simulink model "tr_frame_aided_correlator"  (Simulink 7.9)
settings: Solver=FixedStepDiscrete  SolverMode=SingleTasking  StartTime=0.0  StopTime=120  RelTol=1e-3
undefined symbols (not defined in the file): addr
libraries: shlslibv1 x27
settings Model: synDspstartup=OK  Creator=sszilvasi  LastModifiedBy=sszilvasi
settings DataIOCC: SaveOutput=off  SignalLogging=off  SaveTime=off
settings OptimizationCC: InlineParams=on
settings DebuggingCC: AlgebraicLoopMsg=error  InheritedTsInSrcMsg=none

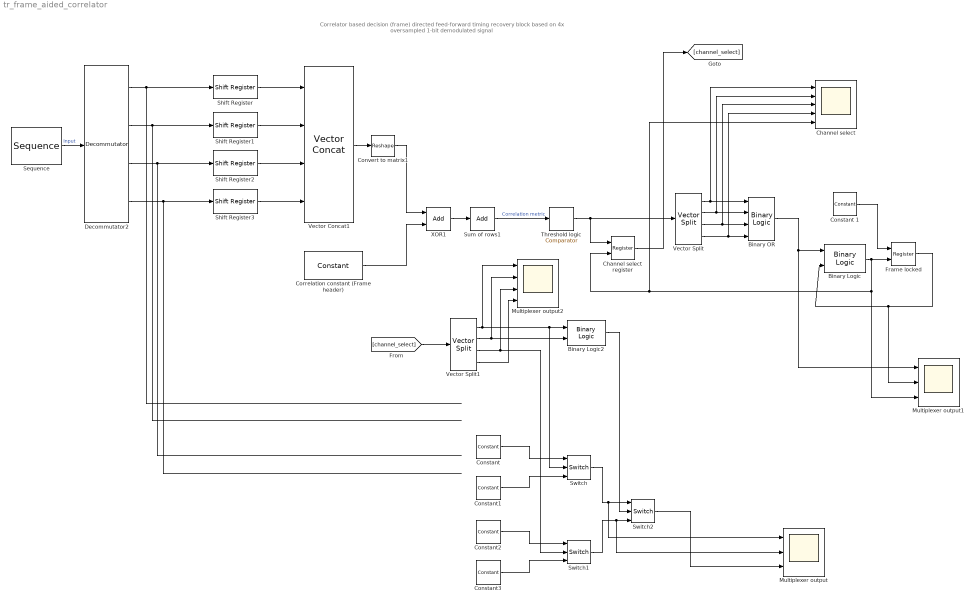
== system tr_frame_aided_correlator ==
  note: Correlator based decision (frame) directed feed-forward timing recovery block
      | based on 4x oversampled 1-bit demodulated signal
  Binary Logic : shlslibv1/Math Functions/Binary Logic  syn_binlog_exp=a&~b  synBlockType=primitive  synLatency=0  synBlockId=13
  Binary Logic2 : shlslibv1/Math Functions/Binary Logic  syn_binlog_exp=a|b  synBlockType=primitive  synLatency=0  synBlockId=13
  Binary OR : shlslibv1/Math Functions/Binary Logic  syn_binlog_exp=a|b|c|d  synBlockType=primitive  synLatency=0  synBlockId=13
  Channel select : Scope  NumInputPorts=5
      settings: YMin=-5~-5~-5~-5~-5  YMax=5~5~5~5~5
  Channel select register : shlslibv1/Memories/Register  syn_delay_val=1  syn_rst_port=off  syn_en_port=on  synBlockType=custom  synLatency=1
  Constant : shlslibv1/Sources/Constant  syn_cst_val=0  syn_cst_fl=0  syn_cst_dt=unsigned  syn_cst_rnd=on  syn_cst_st=-1  synBlockType=primitive  synLatency=0  synBlockId=15
  Constant 1 : shlslibv1/Sources/Constant  syn_cst_val=1  syn_cst_fl=0  syn_cst_dt=unsigned  syn_cst_rnd=on  syn_cst_st=-1  synBlockType=primitive  synLatency=0  synBlockId=15
  Constant1 : shlslibv1/Sources/Constant  syn_cst_val=1  syn_cst_fl=0  syn_cst_dt=unsigned  syn_cst_rnd=on  syn_cst_st=-1  synBlockType=primitive  synLatency=0  synBlockId=15
  Constant2 : shlslibv1/Sources/Constant  syn_cst_val=2  syn_cst_fl=0  syn_cst_dt=unsigned  syn_cst_rnd=on  syn_cst_st=-1  synBlockType=primitive  synLatency=0  synBlockId=15
  Constant3 : shlslibv1/Sources/Constant  syn_cst_val=3  syn_cst_fl=0  syn_cst_dt=unsigned  syn_cst_rnd=on  syn_cst_st=-1  synBlockType=primitive  synLatency=0  synBlockId=15
  Convert to matrix1 : shlslibv1/Signal Operations/Reshape  syn_op_dim_type=Specify  syn_op_dim=[4 4]  syn_ip_order=Column First  syn_op_order=Column First  syn_inh_port=off  synBlockType=primitive  synLatency=0  synBlockId=158
  Correlation constant (Frame header) : shlslibv1/Sources/Constant  syn_cst_val=[1 1 0 0]'*ones(1,4)  syn_cst_fl=0  syn_cst_dt=unsigned  syn_cst_rnd=on  syn_cst_st=-1  synBlockType=primitive  synLatency=0  synBlockId=15
  Decommutator2 : shlslibv1/Signal Operations/Decommutator  syn_outport_nb=4  syn_outport_vec=off  synBlockType=custom  synLatency=1
  Frame locked : shlslibv1/Memories/Register  syn_delay_val=1  syn_rst_port=off  syn_en_port=on  synBlockType=custom  synLatency=1
  Multiplexer output : Scope  NumInputPorts=3
      settings: YMin=-5~-5~-5  YMax=5~5~5
  Multiplexer output1 : Scope  NumInputPorts=3
      settings: YMin=-5~-5~-5  YMax=5~5~5  SaveName=ScopeData2
  Multiplexer output2 : Scope  NumInputPorts=4
      settings: YMin=-5~-5~-5~-5  YMax=5~5~5~5  SaveName=ScopeData3
  Sequence : shlslibv1/Sources/Sequence  syn_seq_vec=[zeros(1,8) 0 0 0 1 1 0 1 0 1]  syn_seq_wl=1  syn_seq_fl=0  syn_seq_dt=unsigned  syn_rst_port=off  syn_en_port=off  syn_seq_st=1  synBlockType=custom  synLatency=1
  Shift Register{,1..3} (4 alike) : shlslibv1/Memories/Shift Register  syn_shift_dynamic=off  syn_shift_vec=[0:3]  syn_shift_val=16  syn_vect_out=Merge to vector  syn_rst_val=All zeros  syn_rst_vec=0  syn_rst_port=off  syn_en_port=off  synBlockType=primitive  synLatency=(addr+1)  synBlockId=93
  Sum of rows1 : shlslibv1/Math Functions/Add  syn_add_opr=+  syn_out_f=Specify  syn_out_wl=3  syn_out_fl=0  syn_out_dt=unsigned  syn_out_sat=off  syn_out_rnd=Floor (Truncate)  synBlockType=primitive  synLatency=0  synBlockId=96  syn_sum_of_rows=on
  Switch : shlslibv1/Signal Operations/Switch  switchCriteria=u2 > Threshold  switchThresh=0  synBlockType=custom  synLatency=0
  Switch1 : shlslibv1/Signal Operations/Switch  switchCriteria=u2 > Threshold  switchThresh=0  synBlockType=custom  synLatency=0
  Switch2 : shlslibv1/Signal Operations/Switch  switchCriteria=u2 > Threshold  switchThresh=0  synBlockType=custom  synLatency=0
  Threshold logic : shlslibv1/Math Functions/Comparator  syn_comp_opr=a==b  syn_comp_const=on  syn_comp_val=0  synBlockType=primitive  synLatency=0  synBlockId=14
  Vector Concat1 : shlslibv1/Signal Operations/Vector Concat  syn_in_nb=4  syn_out_f=Full Precision  syn_out_wl=16  syn_out_fl=8  syn_out_dt=signed  synBlockType=primitive  synLatency=0  synBlockId=19
  Vector Split : shlslibv1/Signal Operations/Vector Split  syn_out_nb=4  synBlockType=primitive  synLatency=0  synBlockId=20
  Vector Split1 : shlslibv1/Signal Operations/Vector Split  syn_out_nb=4  synBlockType=primitive  synLatency=0  synBlockId=20
  XOR1 : shlslibv1/Math Functions/Add  syn_add_opr=++  syn_out_f=Specify  syn_out_wl=1  syn_out_fl=0  syn_out_dt=unsigned  syn_out_sat=off  syn_out_rnd=Floor (Truncate)  synBlockType=primitive  synLatency=0  synBlockId=96  syn_sum_of_rows=off
  wires:
  Sequence/1 -> Decommutator2/1  "Input"
  Decommutator2/1 -> Shift Register/1
  Decommutator2/2 -> Shift Register1/1
  Decommutator2/3 -> Shift Register2/1
  Decommutator2/4 -> Shift Register3/1
  Shift Register/1 -> Vector Concat1/1
  Shift Register1/1 -> Vector Concat1/2
  Shift Register2/1 -> Vector Concat1/3
  Shift Register3/1 -> Vector Concat1/4
  Sum of rows1/1 -> Threshold logic/1  "Correlation metric"
  XOR1/1 -> Sum of rows1/1
  Correlation constant (Frame header)/1 -> XOR1/2
  Vector Concat1/1 -> Convert to matrix1/1
  Convert to matrix1/1 -> XOR1/1
  Vector Split/1 -> Binary OR/1, Channel select/1
  Vector Split/2 -> Binary OR/2, Channel select/2
  Vector Split/3 -> Binary OR/3, Channel select/3
  Vector Split/4 -> Binary OR/4, Channel select/4
  Switch/1 -> Switch2/1, Multiplexer output/1
  Switch1/1 -> Switch2/3, Multiplexer output/2
  Switch2/1 -> Multiplexer output/3
  Binary OR/1 -> Binary Logic/1, Multiplexer output1/1
  Frame locked/1 -> Multiplexer output1/2, Binary Logic/2
  Binary Logic/1 -> Frame locked/2, Multiplexer output1/3, Channel select register/2, Channel select/5
  Constant 1/1 -> Frame locked/1
  Vector Split1/1 -> Switch/2, Binary Logic2/1, Multiplexer output2/1
  Vector Split1/3 -> Switch1/2, Multiplexer output2/3
  Binary Logic2/1 -> Switch2/2
  Constant3/1 -> Switch1/3
  Constant2/1 -> Switch1/1
  Constant1/1 -> Switch/3
  Constant/1 -> Switch/1
  [channel_select] -> Vector Split1/1
  Vector Split1/2 -> Binary Logic2/2, Multiplexer output2/2
  Threshold logic/1 -> Vector Split/1, Channel select register/1
  Channel select register/1 -> [channel_select]
  Vector Split1/4 -> Multiplexer output2/4
